simulink model "testChamberStability"  (R2023b)
settings: Solver=VariableStepAuto  StartTime=0.0  StopTime=10  MaxStep=0.01  MinStep=0.001  RelTol=1e-3
libraries: slident x1, simulink x1
settings Model: Creator=hdt  LastModifiedBy=hdt
settings SolverCC: AutoInsertRateTranBlk=on

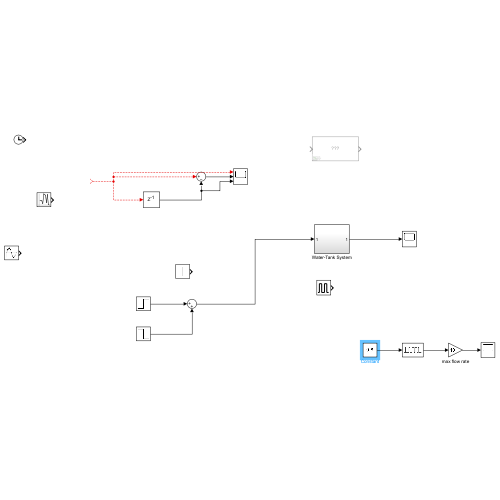
[thumbnail: Simulink's stored preview of the top-level diagram]
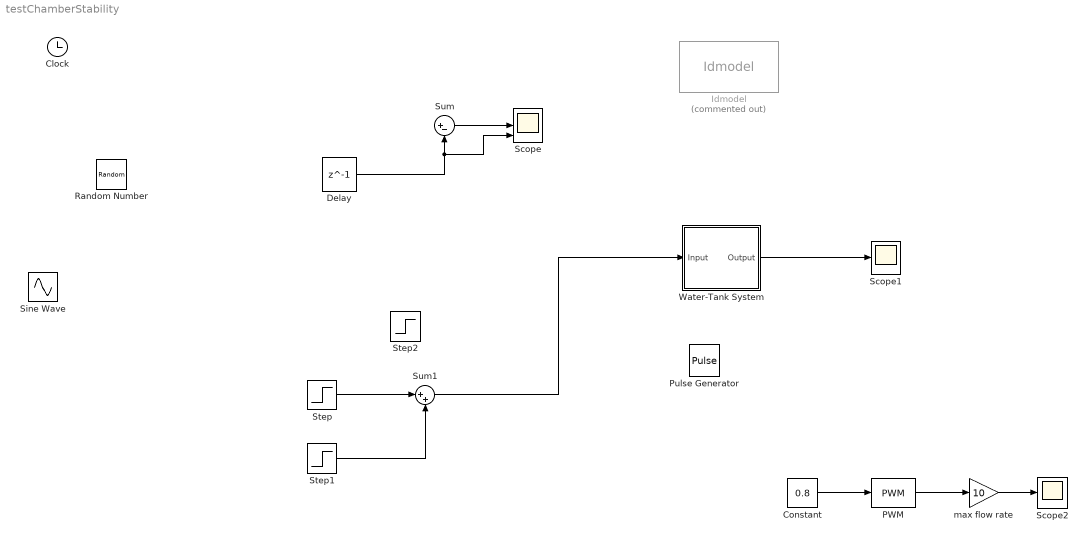
== system testChamberStability ==
  Clock : Clock
  Constant : Constant  Value=0.8
  Delay : Delay  DelayLength=1  SampleTime=1
  Idmodel : slident/Models/Idmodel  Commented=on  sys=chamber  IC=0  noi=off  seed=[]
  PWM : simulink/Discontinuities/PWM  DisableCoverage=on  Period=1  InitialDelay=0  DisallowZeroDutyCycle=off  RunAtFixedTimeIntervals=off  SampleTime=0.1
  Pulse Generator : DiscretePulseGenerator  PulseType=Time based  Period=1200  PulseWidth=25
  Random Number : RandomNumber  Seed=1  SampleTime=1
  Scope : Scope  NumInputPorts=3
  Scope1 : Scope
  Scope2 : Scope
  Sine Wave : Sin  SineType=Sample based  Samples=20  SampleTime=1
  Step : Step  Time=300  SampleTime=0
  Step1 : Step  Time=600  After=-1  SampleTime=0
  Step2 : Step  Time=300  SampleTime=0
  Sum : Sum  Inputs=|+-
  Sum1 : Sum  Inputs=|++
  Water-Tank System : Subsystem
  max flow rate : Gain  Gain=10
  wires:
  Delay/1 -> Scope/3, Sum/2
  Sum/1 -> Scope/2
  ? -> Sum/1, Scope/1, Delay/1
  Water-Tank System/1(Output) -> Scope1/1
  Step1/1 -> Sum1/2
  Step/1 -> Sum1/1
  Sum1/1 -> Water-Tank System/1(Input)
  Constant/1 -> PWM/1
  PWM/1 -> max flow rate/1
  max flow rate/1 -> Scope2/1

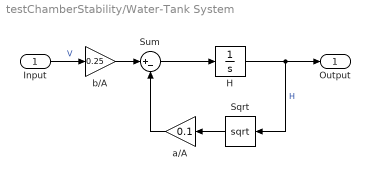
== system testChamberStability/Water-Tank System ==
  Input : Inport
  H : Integrator  LimitOutput=on  LowerSaturationLimit=0
  Sqrt : Sqrt  OutputSignalType=real
  Sum : Sum  Inputs=|+-  SaturateOnIntegerOverflow=on
  a/A : Gain  Gain=0.1  SaturateOnIntegerOverflow=on  OutDataTypeStr=Inherit: Same as input  ParamDataTypeStr=Inherit: Same as input
  b/A : Gain  Gain=0.25  SaturateOnIntegerOverflow=on  OutDataTypeStr=Inherit: Same as input  ParamDataTypeStr=Inherit: Same as input
  Output : Outport  VectorParamsAs1DForOutWhenUnconnected=off
  wires:
  b/A/1 -> Sum/1
  Sum/1 -> H/1
  H/1 -> Sqrt/1, Output/1  "H"
  Sqrt/1 -> a/A/1
  a/A/1 -> Sum/2
  Input/1 -> b/A/1  "V"
